simulink model "IterSubsysEx"  (R2015a)
settings: Solver=FixedStepDiscrete  StartTime=0.0  StopTime=tsim  FixedStep=dt  RelTol=1e-3
values from neighbouring files (symbols this model uses):
  Cp1d = Cp*ones(length(y0),1)'    [run_IterSubsysEx.m]
  hb = 0.03    [run_IterSubsysEx.m]
  ht = 0.03    [run_IterSubsysEx.m]
  k1d = k*ones(length(y0),1)'    [run_IterSubsysEx.m]
  rho1d = rho*ones(length(y0),1)'    [run_IterSubsysEx.m]
  T01d = 550*ones(length(y0),1)'    [run_IterSubsysEx.m]
  Tb = 800    [run_IterSubsysEx.m]
  Tt = 650    [run_IterSubsysEx.m]
libraries: lib_Conduction_HeatX1DVarPropsAndGenBCs_IterSubsysCapable x1, simulink x1
settings Model: Creator=jlkratz  LastModifiedBy=jlkratz

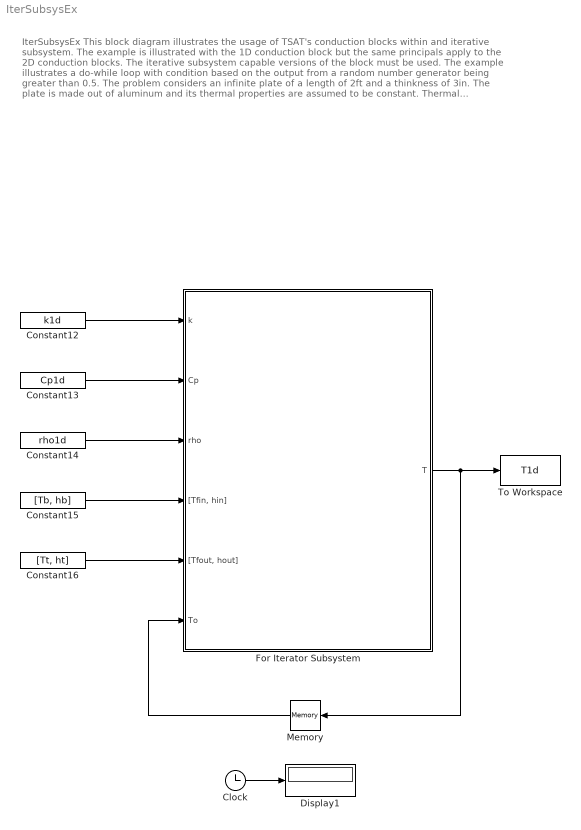
== system IterSubsysEx ==
  note: IterSubsysEx
      |
      | This block diagram illustrates the usage of TSAT's conduction blocks within and iterative subsystem. The example is
      | illustrated with the 1D conduction block but the same principals apply to the 2D conduction blocks. The iterative subsystem
      | capable versions of the block must be used. The example illustrates a do-while loop with condition based on the output
      | from a random number generator being greater than 0.5.
      |
      | The problem considers an infinite plate of a length of 2ft and a thinkness of 3in. The plate is made out of aluminum and
      | its thermal properties are assumed to be constant.
      | Thermal conductivity, k = 0.0328Btu/(sec-ft-R)
      | Heat capacity, Cp = 6.92Btu/(slug-R)
      | Density, rho = 5.24slug/ft^3
      | The plate is at an initial temperature of 550R throughout. It is heated on the bottom surface by convection with a fluid
      | temperature of 800R and heat transfer coefficient of 0.03Btu/(sec-ft^2-R). It is heated on the top surface by convection
      | with a fluid temperature of 650R and heat transfer coefficient of 0.03Btu/(sec-ft^2-R)
  Clock : Clock
  Constant12 : Constant  Value=k1d
  Constant13 : Constant  Value=Cp1d
  Constant14 : Constant  Value=rho1d
  Constant15 : Constant  Value=[Tb, hb]
  Constant16 : Constant  Value=[Tt, ht]
  Display1 : Display
  For Iterator Subsystem : Subsystem  TreatAsAtomicUnit=on
  Memory : Memory  X0=T01d
  To Workspace : ToWorkspace  VariableName=T1d  SaveFormat=Timeseries  SampleTime=-1
  wires:
  Clock/1 -> Display1/1
  For Iterator Subsystem/1(T) -> Memory/1, To Workspace/1
  Memory/1 -> For Iterator Subsystem/6(To)
  Constant12/1 -> For Iterator Subsystem/1(k)
  Constant13/1 -> For Iterator Subsystem/2(Cp)
  Constant14/1 -> For Iterator Subsystem/3(rho)
  Constant15/1 -> For Iterator Subsystem/4("[Tfin, hin]")
  Constant16/1 -> For Iterator Subsystem/5("[Tfout, hout]")

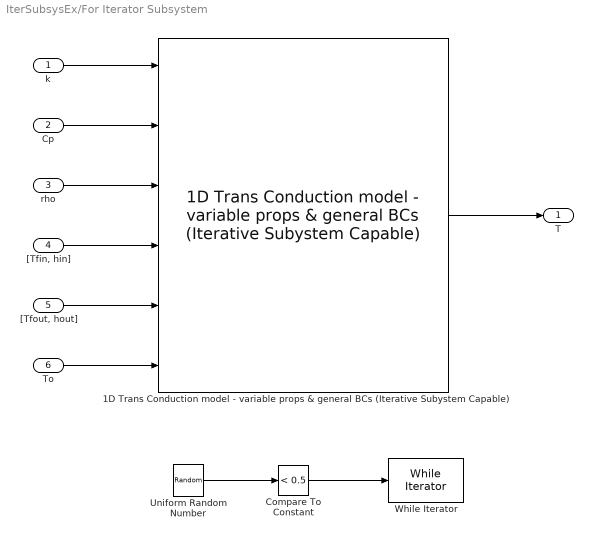
== system IterSubsysEx/For Iterator Subsystem ==
  k : Inport
  Cp : Inport  Port=2
  rho : Inport  Port=3
  "[Tfin, hin]" : Inport  Port=4
  "[Tfout, hout]" : Inport  Port=5
  To : Inport  Port=6
  1D Trans Conduction model - variable props & general BCs (Iterative Subystem Capable) : lib_Conduction_HeatX1DVarPropsAndGenBCs_IterSubsysCapable/1D Trans Conduction model - variable props & general BCs (Iterative Subystem Capable)  x_M=y0  T0_M=T01d  dt_M=dt  a_M=off  convin_M=on  radin_M=off  condin_M=off  convout_M=on  radout_M=off  condout_M=off  BN_M=double(gcb)
  Compare To Constant : simulink/Logic and Bit Operations/Compare To Constant  relop=<  const=0.5  OutDataTypeStr=boolean
  Uniform Random Number : UniformRandomNumber  Minimum=0
  While Iterator : WhileIterator  MaxIters=100  WhileBlockType=do-while
  T : Outport
  wires:
  1D Trans Conduction model - variable props & general BCs (Iterative Subystem Capable)/1 -> T/1
  To/1 -> 1D Trans Conduction model - variable props & general BCs (Iterative Subystem Capable)/6
  k/1 -> 1D Trans Conduction model - variable props & general BCs (Iterative Subystem Capable)/1
  Cp/1 -> 1D Trans Conduction model - variable props & general BCs (Iterative Subystem Capable)/2
  rho/1 -> 1D Trans Conduction model - variable props & general BCs (Iterative Subystem Capable)/3
  "[Tfin, hin]"/1 -> 1D Trans Conduction model - variable props & general BCs (Iterative Subystem Capable)/4
  "[Tfout, hout]"/1 -> 1D Trans Conduction model - variable props & general BCs (Iterative Subystem Capable)/5
  Compare To Constant/1 -> While Iterator/1
  Uniform Random Number/1 -> Compare To Constant/1
